simulink model "Exemplu_figura11"  (R2016a)
settings: Solver=VariableStepDiscrete  StartTime=0.0  StopTime=100  RelTol=1e-3
undefined symbols (not defined in the file): m, n
settings Model: Creator=Cristina  LastModifiedBy=Cristina

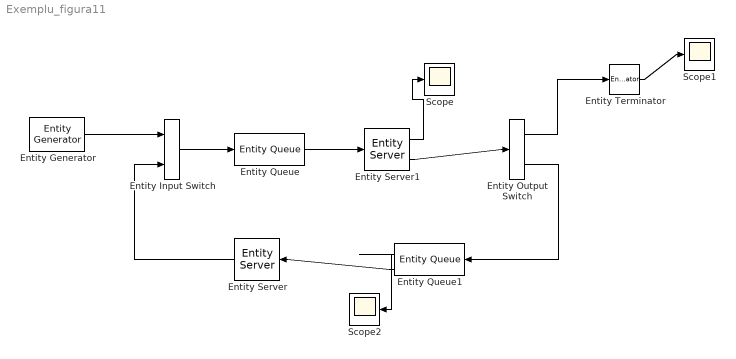
== system Exemplu_figura11 ==
  Entity Input Switch : EntityInputSwitch  InputPortMessageModes=m,m  OutputPortMessageModes=m
  Entity Output Switch : EntityOutputSwitch  InputPortMessageModes=m  OutputPortMessageModes=m,m  SwitchAttributeName=Attribute1
  Entity Generator : EntityGenerator  OutputPortMessageModes=m  TimeSource=MATLAB action  IntergenerationTimeAction=|  EntityType=Structured  EntityTypeName=Entity
      | persistent init
      | if (isemtpy(init))
      |     rng(783);
      |     init = true;
      | end
      | dt = 3.5 + 2 * rand;
  Entity Queue : EntityQueue  InputPortMessageModes=m  OutputPortMessageModes=m
      settings: OutputPortMap=o5
  Entity Queue1 : EntityQueue  InputPortMessageModes=m  OutputPortMessageModes=n,m  NumberEntitiesDeparted=on
      settings: OutputPortMap=o0,o5
  Entity Server : EntityServer  InputPortMessageModes=m  OutputPortMessageModes=m  Capacity=1  ServiceTimeSource=MATLAB action  ServiceTimeAction=|
      | persistent init
      | if (isempty(init))
      |     rng(3737);
      |     init = true;
      | end
      | dt = 20 + 20 * rand;
  Entity Server1 : EntityServer  InputPortMessageModes=m  OutputPortMessageModes=n,m  Capacity=2  ServiceTimeSource=MATLAB action  ServiceTimeAction=|  EntryAction=|  NumberEntitiesInBlock=on
      | persistent init
      | if (isempty(init))
      |     rng(774);
      |     init = true;
      | end;
      | dt = 7 + 6 * rand;
      | persistent init
      | if (isempty(init))
      |     rng(773);
      |     init = true;
      | end
      | if rand < 0.88
      |     entity.PassTest = 1;
      | else
      |     entity.PassTest = 2;
      | end
      settings: OutputPortMap=o1,o9
  Entity Terminator : EntityTerminator  InputPortMessageModes=m  NumberEntitiesArrived=on
      settings: OutputPortMap=o0
  Scope : Scope
  Scope1 : Scope
  Scope2 : Scope
  wires:
  Entity Generator/1 -> Entity Input Switch/1
  Entity Server/1 -> Entity Input Switch/2
  Entity Input Switch/1 -> Entity Queue/1
  Entity Queue/1 -> Entity Server1/1
  Entity Server1/1 -> Scope/1
  Entity Server1/2 -> Entity Output Switch/1
  Entity Output Switch/1 -> Entity Terminator/1
  Entity Terminator/1 -> Scope1/1
  Entity Queue1/2 -> Entity Server/1
  Entity Output Switch/2 -> Entity Queue1/1
  Entity Queue1/1 -> Scope2/1
